simulink model "myproject_task"  (Simulink 3.00)
libraries: mathlib x7, stringlib x3, paramlib x3, speclib x1, genlib x1, matrixlib x1

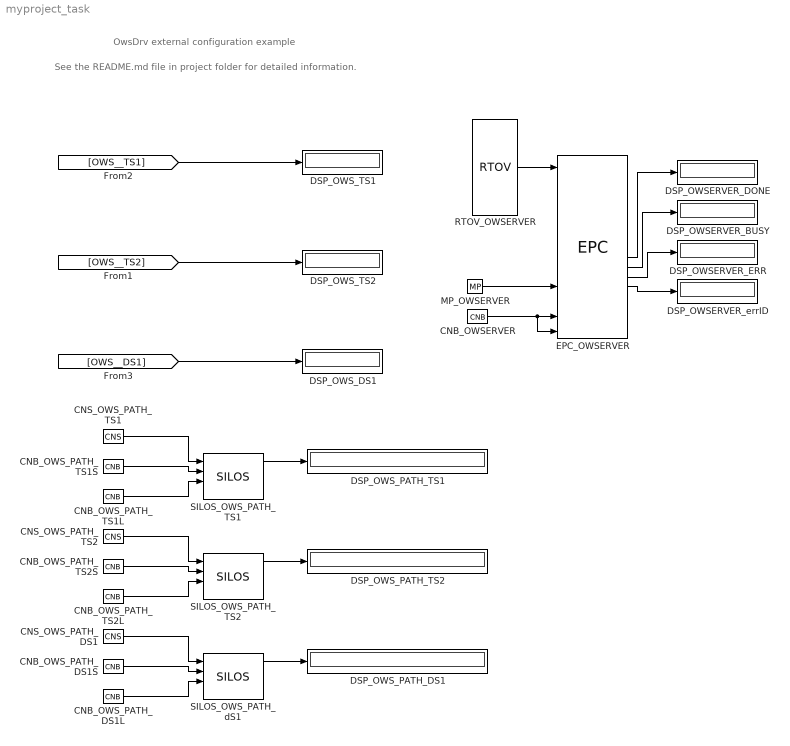
== system myproject_task ==
  note: See the README.md file in project folder for detailed information.
  note: OwsDrv external configuration example
  CNB_OWSERVER : mathlib/CNB  YCN=off
  CNB_OWS_PATH_DS1L : mathlib/CNB  YCN=off
  CNB_OWS_PATH_DS1S : mathlib/CNB  YCN=off
  CNB_OWS_PATH_TS1L : mathlib/CNB  YCN=off
  CNB_OWS_PATH_TS1S : mathlib/CNB  YCN=off
  CNB_OWS_PATH_TS2L : mathlib/CNB  YCN=off
  CNB_OWS_PATH_TS2S : mathlib/CNB  YCN=off
  CNS_OWS_PATH_DS1 : stringlib/CNS  scv=/05.4AEC29CDBAAB = ds1  nmax=22
  CNS_OWS_PATH_TS1 : stringlib/CNS  scv=/28.FFD7816C1403 = ts1  nmax=22
  CNS_OWS_PATH_TS2 : stringlib/CNS  scv=/10.67C6697351FF = ts2  nmax=22
  DSP_OWSERVER_BUSY : Display
      settings: Format=Best fit
  DSP_OWSERVER_DONE : Display
      settings: Format=Best fit
  DSP_OWSERVER_ERR : Display
      settings: Format=Best fit
  DSP_OWSERVER_errID : Display
      settings: Format=Best fit
  DSP_OWS_DS1 : Display
      settings: Format=Best fit
  DSP_OWS_PATH_DS1 : Display
      settings: Format=Best fit
  DSP_OWS_PATH_TS1 : Display
      settings: Format=Best fit
  DSP_OWS_PATH_TS2 : Display
      settings: Format=Best fit
  DSP_OWS_TS1 : Display
      settings: Format=Best fit
  DSP_OWS_TS2 : Display
      settings: Format=Best fit
  EPC_OWSERVER : speclib/EPC  cmd=sudo service owserver restart  sl=0  ifm=1  format=1: Space-delimited values  nmax=2
  MP_OWSERVER : genlib/MP  BSTATE=off  pwidth=2  RPTF=off
  RTOV_OWSERVER : matrixlib/RTOV  nmax=8  offset=0  n=8  etype=8: Double
  SILOS_OWS_PATH_TS1 : paramlib/SILOS  fname=/owfs/ow-ts1  CSF=off  CLF=off  LLO=off  nmax=0
  SILOS_OWS_PATH_TS2 : paramlib/SILOS  fname=/owfs/ow-ts2  CSF=off  CLF=off  LLO=off  nmax=0
  SILOS_OWS_PATH_dS1 : paramlib/SILOS  fname=/owfs/ow-ds1  CSF=off  CLF=off  LLO=off  nmax=0
  wires:
  CNB_OWSERVER/1 -> EPC_OWSERVER/11, EPC_OWSERVER/12
  CNB_OWS_PATH_DS1L/1 -> SILOS_OWS_PATH_dS1/3
  CNB_OWS_PATH_DS1S/1 -> SILOS_OWS_PATH_dS1/2
  CNB_OWS_PATH_TS1L/1 -> SILOS_OWS_PATH_TS1/3
  CNB_OWS_PATH_TS1S/1 -> SILOS_OWS_PATH_TS1/2
  CNB_OWS_PATH_TS2L/1 -> SILOS_OWS_PATH_TS2/3
  CNB_OWS_PATH_TS2S/1 -> SILOS_OWS_PATH_TS2/2
  CNS_OWS_PATH_DS1/1 -> SILOS_OWS_PATH_dS1/1
  CNS_OWS_PATH_TS1/1 -> SILOS_OWS_PATH_TS1/1
  CNS_OWS_PATH_TS2/1 -> SILOS_OWS_PATH_TS2/1
  EPC_OWSERVER/9 -> DSP_OWSERVER_DONE/1
  EPC_OWSERVER/10 -> DSP_OWSERVER_BUSY/1
  EPC_OWSERVER/11 -> DSP_OWSERVER_ERR/1
  EPC_OWSERVER/12 -> DSP_OWSERVER_errID/1
  [OWS__TS2] -> DSP_OWS_TS2/1
  [OWS__TS1] -> DSP_OWS_TS1/1
  [OWS__DS1] -> DSP_OWS_DS1/1
  MP_OWSERVER/1 -> EPC_OWSERVER/9
  RTOV_OWSERVER/1 -> EPC_OWSERVER/1
  SILOS_OWS_PATH_TS1/1 -> DSP_OWS_PATH_TS1/1
  SILOS_OWS_PATH_TS2/1 -> DSP_OWS_PATH_TS2/1
  SILOS_OWS_PATH_dS1/1 -> DSP_OWS_PATH_DS1/1
